simulink subsystem "WindGFLMpp"  (R2025b)
settings: Solver=VariableStepAuto  StartTime=0.0  StopTime=10.0  RelTol=1e-3
model mask{p=0, psim=0, Rs=0, Ld=0, Lq=0, Kdip_sm=0, Kdii_sm=0, Kqip_sm=0, Kqii_sm=0, airDensity=0, turbineRadius=0, pitch=0, TSR=0, cp=0, wt=0, rt=0, Inertia=0, Kp_dc=0, Ki_dc=0, Kdpi_g=0, Kdii_g=0, Kqpi_g=0, Kqii_g=0, blk=Enabled, slop=0, tst=0}
  mask prompts: p "Number of pole pairs"; psim "PMSM flux linkage"; Rs "Stator resistance (Ohms)"; Ld "Stator d-axis inductance (H)"; Lq "Stator q-axis inductance (H)"; Kdip_sm "d-axis proportional gain"; Kdii_sm "d-axis integral gain"; Kqip_sm "q-axis proportional gain"; Kqii_sm "q-axis integral gain"; airDensity "Air Density"; turbineRadius "Turbine radius"; pitch "Pitch angle vector"; cp "Power Coefficient (cp)"; wt "Wind velocity threshold"; rt "Rotational velocity threshold"; Inertia "Turbine Inertia (kgm^2)"; Kp_dc "Proportional gain"; Ki_dc "Integral gain"; Kdpi_g "d-axis proportional gain"; Kdii_g "d-axis integrall gain"; Kqpi_g "q-axis proportional gain"; Kqii_g "q-axis integral gain"; blk "Enable Black Start"; slop "Power Ramp Slope"; tst "Black Start time (sec)"
undefined symbols (not defined in the file): base, DiscIntNeverNeededParam, grid, mpptPower, mpptWindSpeed, Ts, windController, windInverter, windTurbine
libraries: nesl_utility x13, ee_lib x8, fl_lib x8, simulink x6, eeTransforms x4, eeGeneralControl x1, eePmsmCurrentController x1
settings Model: Creator=rajarshd  LastModifiedBy=rajarshd
settings OptimizationCC: ReuseModelBlockBuffer=off
settings RTWCC: GPUComputeCapability=3.5

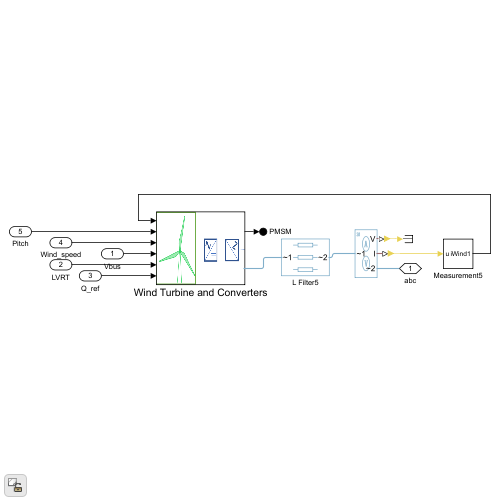
[thumbnail: Simulink's stored preview of the top-level diagram]
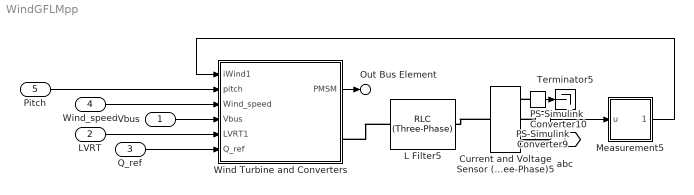
== system WindGFLMpp ==
  Vbus : Inport
  LVRT : Inport  Port=2
  Q_ref : Inport  Port=3
  Wind_speed : Inport  Port=4
  Pitch : Inport  Port=5
  Current and Voltage Sensor (Three-Phase)5 : ee_lib/Sensors & Transducers/Current and Voltage Sensor (Three-Phase)  vMeasurementType=ee.enum.vmeasurement.lg  outputUnit=ee.enum.unit.pu  SRated=base.mVA A*V  VRated=base.kV V  I_specify=off  I_priority=None  I=[0, 0, 0] A  I_nominal_specify=off  I_nominal_value=1  I_nominal_unit=A  V_specify=off  V_priority=None  V=[0, 0, 0] V  V_nominal_specify=off  V_nominal_value=1  V_nominal_unit=V
      settings: InternalSimscapePortConfiguration="{\"Bottom\":[],\"Left\":[{\"id\":\"N1\",\"label\":\"~1\",\"type\":\"foundation.electrical.three_phase\"}],\"Right\":[{\"id\":\"V_output\",\"label\":\"V\",\"type\":\"output\"},{\"id\":\"I_output\",\"label\":\"I\",\"type\":\"output\"},{\"id\":\"N2\",\"label\":\"~2\",\"type\":\"foundation.electrical.three_phase\"}],\"Top\":[]}"
  L Filter5 : ee_lib/Passive/RLC Assemblies/RLC (Three-Phase)  port_option=ee.enum.threePhasePort.composite  component_structure=ee.enum.rlc.structure.L  R=1e-3 Ohm  L=windInverter.l H  C=1e-6 F  R_parasitic=0 Ohm  G_parasitic=0 1/Ohm  IL_specify=off  IL_priority=High  IL=[0, 0, 0] A  IL_nominal_specify=off  IL_nominal_value=1  IL_nominal_unit=A  VC_specify=off  VC_priority=High  VC=[0, 0, 0] V  VC_nominal_specify=off  VC_nominal_value=1  VC_nominal_unit=V
      settings: InternalSimscapePortConfiguration="{\"Bottom\":[],\"Left\":[{\"id\":\"N1\",\"label\":\"~1\",\"type\":\"foundation.electrical.three_phase\"}],\"Right\":[{\"id\":\"N2\",\"label\":\"~2\",\"type\":\"foundation.electrical.three_phase\"}],\"Top\":[]}"
  Measurement5 : Subsystem
  PS-Simulink Converter10 : nesl_utility/PS-Simulink Converter  PhysicalDomain=network_engine_domain  SubClassName=ps_output  LeftPortType=input  RightPortType=output  PseudoPeriodic=off  Frequencies=[]  VectorFormat=inherit  Unit=inherit  AffineConversion=off
  PS-Simulink Converter9 : nesl_utility/PS-Simulink Converter  PhysicalDomain=network_engine_domain  SubClassName=ps_output  LeftPortType=input  RightPortType=output  PseudoPeriodic=off  Frequencies=[]  VectorFormat=inherit  Unit=inherit  AffineConversion=off
  Terminator5 : Terminator
  Wind Turbine and Converters : Subsystem
      mask Display: image('T4wind.png'); % Use "Edit Image" on toolstrip to change.
  abc : PMIOPort  Side=Right
  Out Bus Element : Outport  PortName=PMSM
  wires:
  PS-Simulink Converter10/1 -> Terminator5/1
  PS-Simulink Converter9/1 -> Measurement5/1(u)
  Wind_speed/1 -> Wind Turbine and Converters/3(Wind_speed)
  Wind Turbine and Converters/1(PMSM) -> Out Bus Element/1
  Vbus/1 -> Wind Turbine and Converters/4(Vbus)
  LVRT/1 -> Wind Turbine and Converters/5(LVRT1)
  Q_ref/1 -> Wind Turbine and Converters/6(Q_ref)
  Measurement5/1(iWind1) -> Wind Turbine and Converters/1(iWind1)
  Pitch/1 -> Wind Turbine and Converters/2(pitch)
  connections:
  PS-Simulink Converter9/LConn1 -- Current and Voltage Sensor (Three-Phase)5/RConn2
  PS-Simulink Converter10/LConn1 -- Current and Voltage Sensor (Three-Phase)5/RConn1
  L Filter5/LConn1 -- Wind Turbine and Converters/RConn1
  Current and Voltage Sensor (Three-Phase)5/LConn1 -- L Filter5/RConn1
  Current and Voltage Sensor (Three-Phase)5/RConn3 -- abc/RConn1

== system WindGFLMpp/Measurement5 ==
  u : Inport
  Low-Pass Filter (Discrete or Continuous) : eeGeneralControl/Low-Pass Filter (Discrete or Continuous)  K=1  T=2e-4  B=inf  A=-inf  init_option=Inherited from block input  x0=0  Ts=-1
  Out Bus Element : Outport  PortName=iWind1  Element=1
  wires:
  Low-Pass Filter (Discrete or Continuous)/1 -> Out Bus Element/1
  u/1 -> Low-Pass Filter (Discrete or Continuous)/1

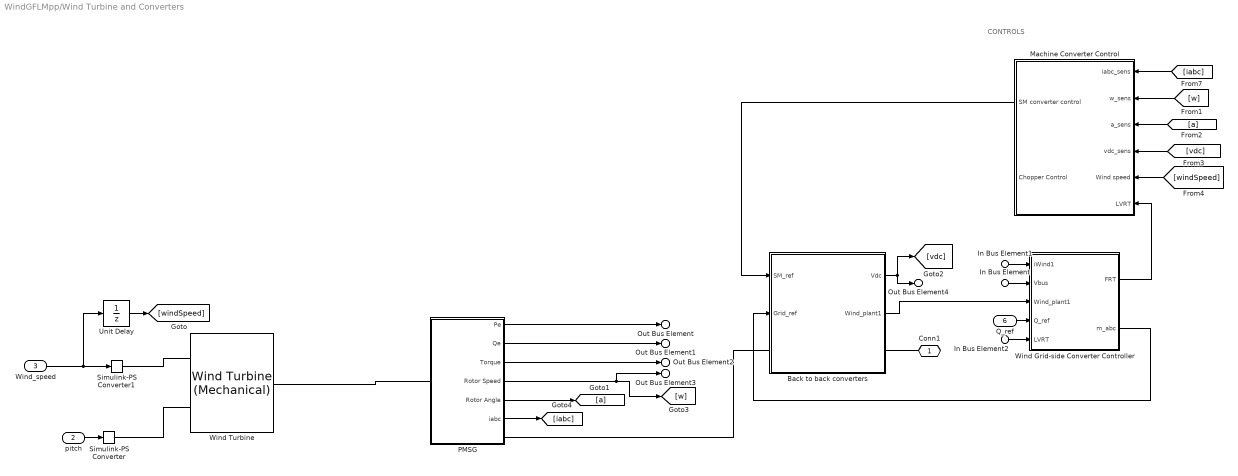
== system WindGFLMpp/Wind Turbine and Converters ==
  note: CONTROLS
  In Bus Element1 : Inport  PortName=iWind1
  pitch : Inport  Port=2
  Wind_speed : Inport  Port=3
  In Bus Element : Inport  Port=4  PortName=Vbus
  In Bus Element2 : Inport  Port=5  PortName=LVRT1
  Q_ref : Inport  Port=6
  Back to back converters : Subsystem
  Machine Converter Control : Subsystem
  PMSG : Subsystem
  Simulink-PS Converter : nesl_utility/Simulink-PS Converter  PhysicalDomain=network_engine_domain  SubClassName=ps_input  LeftPortType=input  RightPortType=output  PseudoPeriodic=off  Frequencies=[]  NoiseDistribution=none  NoiseParameters=[]  Unit=1  AffineConversion=off  FilteringAndDerivatives=provide  SimscapeFilterOrder=1  InputFilterTimeConstant=0.001  UdotUserProvided=0
  Simulink-PS Converter1 : nesl_utility/Simulink-PS Converter  PhysicalDomain=network_engine_domain  SubClassName=ps_input  LeftPortType=input  RightPortType=output  PseudoPeriodic=off  Frequencies=[]  NoiseDistribution=none  NoiseParameters=[]  Unit=1  AffineConversion=off  FilteringAndDerivatives=provide  SimscapeFilterOrder=1  InputFilterTimeConstant=0.001  UdotUserProvided=0
  Unit Delay : UnitDelay  SampleTime=-1  HasFrameUpgradeWarning=on
  Wind Grid-side Converter Controller : Subsystem
  "Wind Turbine " : ee_lib/Electromechanical/Wind Turbine (Mechanical)  R_rotor=turbineRadius m  pitch_TLU=pitch deg  lambda_TLU=TSR  Cp_TLU=cp  v_thr=wt m/s  w_thr=rt rad/s  rho_air=airDensity kg/m^3  includeInertia=true  J=Inertia kg*m^2  lam=0 N*m*s/rad  w_specify=off  w_priority=Low  w=2.262*2.5 rad/s  w_nominal_specify=off  w_nominal_value=1  w_nominal_unit=rad/s  t_specify=off  t_priority=None  t=0 N*m  t_nominal_specify=off  t_nominal_value=1  t_nominal_unit=N*m  Torque_specify=off  Torque_priority=None  Torque=0 N*m  Torque_nominal_specify=off  Torque_nominal_value=1  Torque_nominal_unit=N*m
      settings: InternalSimscapePortConfiguration="{\"Bottom\":[],\"Left\":[{\"id\":\"vWind\",\"label\":\"V\",\"type\":\"input\"},{\"id\":\"pitch\",\"label\":\"β\",\"type\":\"input\"}],\"Right\":[{\"id\":\"R\",\"label\":\"R\",\"type\":\"foundation.mechanical.rotational.rotational\"}],\"Top\":[]}"
  Conn1 : PMIOPort  Side=Right
  Out Bus Element : Outport  PortName=PMSM  Element=P
  Out Bus Element1 : Outport  PortName=PMSM  Element=Q
  Out Bus Element2 : Outport  PortName=PMSM  Element=Torque
  Out Bus Element3 : Outport  PortName=PMSM  Element=w_speed
  Out Bus Element4 : Outport  PortName=PMSM  Element=Vdc
  wires:
  Wind Grid-side Converter Controller/2(m_abc) -> Back to back converters/2(Grid_ref)
  Machine Converter Control/1(SM converter control) -> Back to back converters/1(SM_ref)
  In Bus Element2/1 -> Wind Grid-side Converter Controller/5(LVRT)
  Back to back converters/2(Wind_plant1) -> Wind Grid-side Converter Controller/3(Wind_plant1)
  Q_ref/1 -> Wind Grid-side Converter Controller/4(Q_ref)
  Wind Grid-side Converter Controller/1(FRT) -> Machine Converter Control/6(LVRT)
  In Bus Element/1 -> Wind Grid-side Converter Controller/2(Vbus)
  PMSG/1(Pe) -> Out Bus Element/1
  PMSG/5(Rotor Angle) -> [a]
  Back to back converters/1(Vdc) -> Out Bus Element4/1, [vdc]
  PMSG/6(iabc) -> [iabc]
  pitch/1 -> Simulink-PS Converter/1
  [windSpeed] -> Machine Converter Control/5(Wind speed)
  [w] -> Machine Converter Control/2(w_sens)
  [a] -> Machine Converter Control/3(a_sens)
  Wind_speed/1 -> Unit Delay/1, Simulink-PS Converter1/1
  [iabc] -> Machine Converter Control/1(iabc_sens)
  Unit Delay/1 -> [windSpeed]
  [vdc] -> Machine Converter Control/4(vdc_sens)
  In Bus Element1/1 -> Wind Grid-side Converter Controller/1(iWind1)
  PMSG/3(Torque) -> Out Bus Element2/1
  PMSG/2(Qe) -> Out Bus Element1/1
  PMSG/4(Rotor Speed) -> Out Bus Element3/1, [w]
  connections:
  PMSG/RConn1 -- Back to back converters/LConn1
  Conn1/RConn1 -- Back to back converters/RConn1
  "Wind Turbine "/LConn1 -- Simulink-PS Converter1/RConn1
  "Wind Turbine "/LConn2 -- Simulink-PS Converter/RConn1
  "Wind Turbine "/RConn1 -- PMSG/LConn1

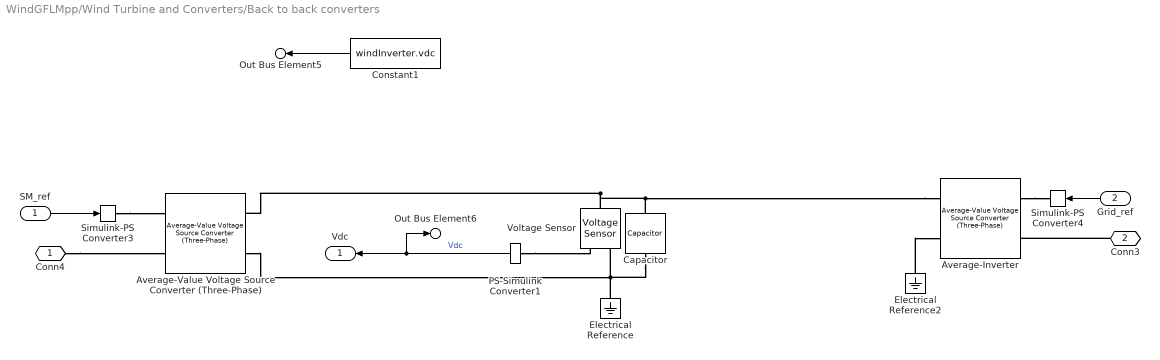
== system WindGFLMpp/Wind Turbine and Converters/Back to back converters ==
  SM_ref : Inport
  Grid_ref : Inport  Port=2
  Average-Inverter : ee_lib/Semiconductors & Converters/Converters/Average-Value Voltage Source Converter (Three-Phase)  port_option=ee.enum.threePhasePort.composite  frequency_option=ee.enum.converters.frequency.variable  input_option=ee.enum.converters.inputOption.ModWave  FRated=60 Hz  losses_parameterization=ee.enum.converters.losses.fixed  Pfixed=1 W  ks=0.01  kc1=1.7 V  kc2=0.01 Ohm  Ploss_vect=[100, 800, 1870, 3250, 4900] W  Irms_vect=[10, 100, 200, 300, 400] A  Vdc_nom=300 V  thermal_mass=30000 J/K  temperature_specify=off  temperature_priority=High  temperature=298.15 K  temperature_nominal_specify=off  temperature_nominal_value=1  temperature_nominal_unit=K
      settings: InternalSimscapePortConfiguration="{\"Bottom\":[],\"Left\":[{\"id\":\"ModWave\",\"label\":\"ModWave\",\"type\":\"input\"},{\"id\":\"N\",\"label\":\"~\",\"type\":\"foundation.electrical.three_phase\"}],\"Right\":[{\"id\":\"p\",\"label\":\"+\",\"type\":\"foundation.electrical.electrical\"},{\"id\":\"n\",\"label\":\"-\",\"type\":\"foundation.electrical.electrical\"}],\"Top\":[]}"
  Average-Value Voltage Source Converter (Three-Phase) : ee_lib/Semiconductors & Converters/Converters/Average-Value Voltage Source Converter (Three-Phase)  port_option=ee.enum.threePhasePort.composite  frequency_option=ee.enum.converters.frequency.variable  input_option=ee.enum.converters.inputOption.ModWave  FRated=60 Hz  losses_parameterization=ee.enum.converters.losses.fixed  Pfixed=1 W  ks=0.01  kc1=1.7 V  kc2=0.01 Ohm  Ploss_vect=[100, 800, 1870, 3250, 4900] W  Irms_vect=[10, 100, 200, 300, 400] A  Vdc_nom=300 V  thermal_mass=30000 J/K  temperature_specify=off  temperature_priority=High  temperature=298.15 K  temperature_nominal_specify=off  temperature_nominal_value=1  temperature_nominal_unit=K
      settings: InternalSimscapePortConfiguration="{\"Bottom\":[],\"Left\":[{\"id\":\"ModWave\",\"label\":\"ModWave\",\"type\":\"input\"},{\"id\":\"N\",\"label\":\"~\",\"type\":\"foundation.electrical.three_phase\"}],\"Right\":[{\"id\":\"p\",\"label\":\"+\",\"type\":\"foundation.electrical.electrical\"},{\"id\":\"n\",\"label\":\"-\",\"type\":\"foundation.electrical.electrical\"}],\"Top\":[]}"
  Capacitor : fl_lib/Electrical/Electrical Elements/Capacitor  c=windInverter.c F  r=0 Ohm  g=0 1/Ohm  i_specify=off  i_priority=None  i=0 A  i_nominal_specify=off  i_nominal_value=1  i_nominal_unit=A  v_specify=off  v_priority=None  v=0 V  v_nominal_specify=off  v_nominal_value=1  v_nominal_unit=V  vc_specify=on  vc_priority=Low  vc=windInverter.vdc V  vc_nominal_specify=off  vc_nominal_value=1  vc_nominal_unit=V
  Constant1 : Constant  Value=windInverter.vdc  SampleTime=Ts
  Electrical Reference : fl_lib/Electrical/Electrical Elements/Electrical Reference
  Electrical Reference2 : fl_lib/Electrical/Electrical Elements/Electrical Reference
  PS-Simulink Converter1 : nesl_utility/PS-Simulink Converter  PhysicalDomain=network_engine_domain  SubClassName=ps_output  LeftPortType=input  RightPortType=output  PseudoPeriodic=off  Frequencies=[]  VectorFormat=1-D array  Unit=V  AffineConversion=off
  Simulink-PS Converter3 : nesl_utility/Simulink-PS Converter  PhysicalDomain=network_engine_domain  SubClassName=ps_input  LeftPortType=input  RightPortType=output  PseudoPeriodic=off  Frequencies=[]  NoiseDistribution=none  NoiseParameters=[]  Unit=1  AffineConversion=off  FilteringAndDerivatives=provide  SimscapeFilterOrder=1  InputFilterTimeConstant=0.001  UdotUserProvided=0
  Simulink-PS Converter4 : nesl_utility/Simulink-PS Converter  PhysicalDomain=network_engine_domain  SubClassName=ps_input  LeftPortType=input  RightPortType=output  PseudoPeriodic=off  Frequencies=[]  NoiseDistribution=none  NoiseParameters=[]  Unit=1  AffineConversion=off  FilteringAndDerivatives=provide  SimscapeFilterOrder=1  InputFilterTimeConstant=0.001  UdotUserProvided=0
  Voltage Sensor : fl_lib/Electrical/Electrical Sensors/Voltage Sensor
  Conn4 : PMIOPort  Side=Left
  Conn3 : PMIOPort  Port=2  Side=Right
  Vdc : Outport
  Out Bus Element6 : Outport  Port=2  PortName=Wind_plant1  Element=Vdc_measured
  Out Bus Element5 : Outport  Port=2  PortName=Wind_plant1  Element=windInverter.vdc
  wires:
  Constant1/1 -> Out Bus Element5/1
  SM_ref/1 -> Simulink-PS Converter3/1
  Grid_ref/1 -> Simulink-PS Converter4/1
  PS-Simulink Converter1/1 -> Vdc/1, Out Bus Element6/1  "Vdc"
  connections:
  Conn3/RConn1 -- Average-Inverter/LConn2
  Simulink-PS Converter3/RConn1 -- Average-Value Voltage Source Converter (Three-Phase)/LConn1
  Average-Inverter/LConn1 -- Simulink-PS Converter4/RConn1
  Conn4/RConn1 -- Average-Value Voltage Source Converter (Three-Phase)/LConn2
  Average-Value Voltage Source Converter (Three-Phase)/RConn2 -- Electrical Reference/LConn1 -- Capacitor/RConn1 -- Voltage Sensor/RConn2
  Electrical Reference2/LConn1 -- Average-Inverter/RConn2
  Average-Inverter/RConn1 -- Capacitor/LConn1 -- Average-Value Voltage Source Converter (Three-Phase)/RConn1 -- Voltage Sensor/LConn1
  PS-Simulink Converter1/LConn1 -- Voltage Sensor/RConn1

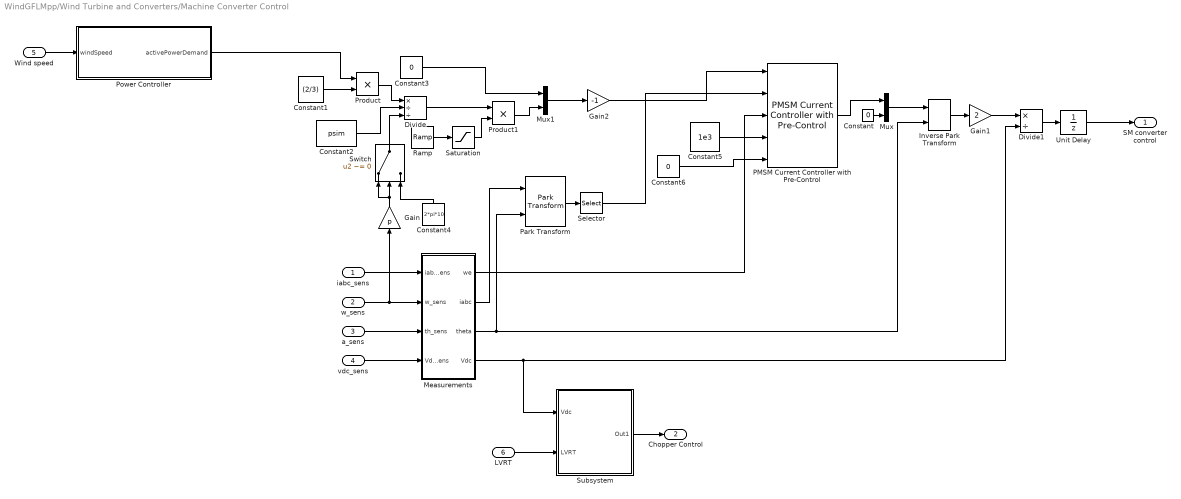
== system WindGFLMpp/Wind Turbine and Converters/Machine Converter Control ==
  iabc_sens : Inport
  w_sens : Inport  Port=2
  a_sens : Inport  Port=3
  vdc_sens : Inport  Port=4
  Wind speed : Inport  Port=5
  LVRT : Inport  Port=6
  Constant : Constant  Value=0  SampleTime=-1
  Constant1 : Constant  Value=(2/3)
  Constant2 : Constant  Value=psim
  Constant3 : Constant  Value=0
  Constant4 : Constant  Value=2*pi*10
  Constant5 : Constant  Value=1e3  VectorParams1D=off  SampleTime=-1
  Constant6 : Constant  Value=0
  Divide : Product  Inputs=*//
  Divide1 : Product  Inputs=*/
  Gain : Gain  Gain=p
  Gain1 : Gain  Gain=2
  Gain2 : Gain  Gain=-1
  Inverse Park Transform : eeTransforms/Inverse Park Transform  AxisAlignment=Q-axis  PowerInvariant=off
  Measurements : Subsystem
  Mux : Mux  Inputs=2
  Mux1 : Mux  Inputs=2
  PMSM Current Controller with Pre-Control : eePmsmCurrentController/PMSM Current Controller with Pre-Control  Kp_id=Kdip_sm  Ki_id=Kdii_sm  Kaw_id=0  Kp_iq=Kqip_sm  Ki_iq=Kqii_sm  Kaw_iq=0  Ts=-1  Tsd=0.001  AxisPrio=Q-axis  ActZC=off  ActFF=on  idVect=[-1, 0, 1]  iqVect=[-2000, 0, 2000]  LdMatrix=Ld* ones(3, 3)  LqMatrix=Lq* ones(3, 3)  psimMatrix=psim * ones(3, 3)
  Park Transform : eeTransforms/Park Transform  AxisAlignment=Q-axis  PowerInvariant=off
  Power Controller : Subsystem
  Product : Product
  Product1 : Product
  Ramp : simulink/Sources/Ramp  slope=slop  start=tst  InitialOutput=blk
  Saturation : Saturate  UpperLimit=1  LowerLimit=0
  Selector : Selector  InputPortWidth=3  IndexOptions=Index vector (dialog)  Indices=[1 2]  OutputSizes=1
  Subsystem : Subsystem
  Switch : Switch  Criteria=u2 ~= 0  SaturateOnIntegerOverflow=off  InputSameDT=off
  Unit Delay : UnitDelay  SampleTime=-1  HasFrameUpgradeWarning=on
  SM converter control : Outport  VectorParamsAs1DForOutWhenUnconnected=off
  Chopper Control : Outport  Port=2
  wires:
  Saturation/1 -> Product1/2
  Product1/1 -> Mux1/2
  Divide/1 -> Product1/1
  Power Controller/1(activePowerDemand) -> Product/1
  Ramp/1 -> Saturation/1
  Wind speed/1 -> Power Controller/1(windSpeed)
  Subsystem/1(Out1) -> Chopper Control/1
  LVRT/1 -> Subsystem/2(LVRT)
  PMSM Current Controller with Pre-Control/1 -> Mux/1
  Gain2/1 -> PMSM Current Controller with Pre-Control/1
  Constant4/1 -> Switch/3
  Switch/1 -> Divide/3
  Gain/1 -> Switch/2, Switch/1
  Constant1/1 -> Product/2
  Product/1 -> Divide/1
  Mux1/1 -> Gain2/1
  Constant3/1 -> Mux1/1
  Constant2/1 -> Divide/2
  Constant6/1 -> PMSM Current Controller with Pre-Control/5
  Constant5/1 -> PMSM Current Controller with Pre-Control/4
  Gain1/1 -> Divide1/1
  Selector/1 -> PMSM Current Controller with Pre-Control/2
  Park Transform/1 -> Selector/1
  Measurements/3(theta) -> Inverse Park Transform/2, Park Transform/2
  Measurements/2(iabc) -> Park Transform/1
  Unit Delay/1 -> SM converter control/1
  Constant/1 -> Mux/2
  Mux/1 -> Inverse Park Transform/1
  Inverse Park Transform/1 -> Gain1/1
  a_sens/1 -> Measurements/3(th_sens)
  iabc_sens/1 -> Measurements/1(iabc_sens)
  Measurements/1(we) -> PMSM Current Controller with Pre-Control/3
  w_sens/1 -> Measurements/2(w_sens), Gain/1
  vdc_sens/1 -> Measurements/4(Vdc_sens)
  Divide1/1 -> Unit Delay/1
  Measurements/4(Vdc) -> Divide1/2, Subsystem/1(Vdc)

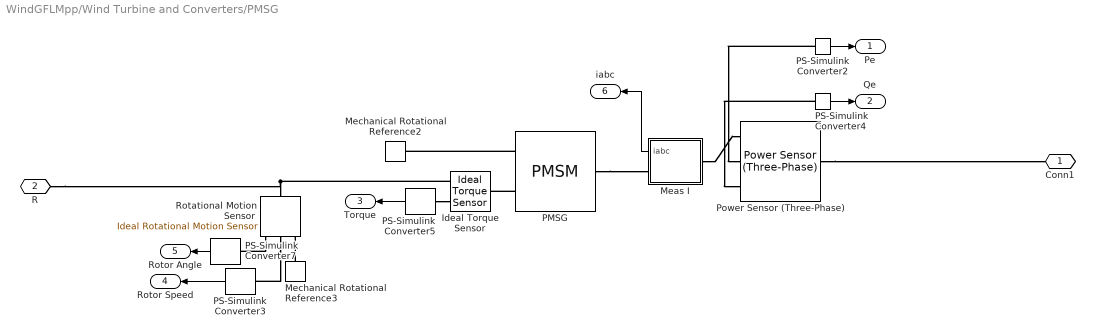
== system WindGFLMpp/Wind Turbine and Converters/PMSG ==
  Ideal Torque Sensor : fl_lib/Mechanical/Mechanical Sensors/Ideal Torque Sensor
  Meas I : Subsystem
  Mechanical Rotational Reference2 : fl_lib/Mechanical/Rotational Elements/Mechanical Rotational Reference
  Mechanical Rotational Reference3 : fl_lib/Mechanical/Rotational Elements/Mechanical Rotational Reference
  PMSG : ee_lib/Electromechanical/Permanent Magnet/PMSM  port_option=ee.enum.threePhasePort.composite  winding_type=ee.enum.statorconnection.wye  machine_param=ee.enum.pmsm.parameterization.constant  nPolePairs=p  pmflux_param=ee.enum.pmflux.fluxlinkage  pm_flux_linkage=psim Wb  torque_constant=0.18 N*m/A  back_emf_constant=0.18 V*s/rad  stator_param=ee.enum.statorparam.LdLqL0  Ld=Ld H  Lq=Lq H  idVec=[-200, 0, 200] A  iqVec=[-200, 0, 200] A  LdMatrix=0.0002 * ones(3, 3) H  LqMatrix=0.0002 * ones(3, 3) H  PmMatrix=0.1 * ones(3, 3) Wb  ktMatrix=0.18 * ones(3, 3) N*m/A  keMatrix=0.18 * ones(3, 3) V*s/rad  L0=0.00016 H  Ls=0.0002 H  Lm=-0.00002 H  Ms=0.00002 H  Rs=Rs Ohm  zero_sequence=ee.enum.park.zerosequence.exclude  axes_param=ee.enum.rotorangle.qaxis  loss_param=ee.enum.ironloss.none  losses_oc=[0, 0, 0] W  losses_sc=[0, 0, 0] W  f_losses=60 Hz  Isc_losses=95 A  J=200 kg*m^2  lam=1e-4 N*m*s/rad  i_d_specify=off  i_d_priority=None  i_d=0 A  i_d_nominal_specify=off  i_d_nominal_value=1  i_d_nominal_unit=A  i_q_specify=off  i_q_priority=None  i_q=0 A  i_q_nominal_specify=off  i_q_nominal_value=1  i_q_nominal_unit=A  torque_specify=off  torque_priority=None  torque=0 N*m  torque_nominal_specify=off  torque_nominal_value=1  torque_nominal_unit=N*m  angular_velocity_specify=on  angular_velocity_priority=High  angular_velocity=2.26 rad/s  angular_velocity_nominal_specify=off  angular_velocity_nominal_value=1  angular_velocity_nominal_unit=rpm  angular_position_specify=off  angular_position_priority=High  angular_position=0 deg  angular_position_nominal_specify=off  angular_position_nominal_value=1  angular_position_nominal_unit=deg  alpha=3.93e-3 1/K  alpha_flux=-0.001 1/K  Tmeas=298.15 K  stator_thermal_mass=100 J/K  rotor_thermal_mass=200 J/K  Rm_percent_rotor=90  Rd_percent_rotor=30  temperatureA_specify=off  temperatureA_priority=High  temperatureA=25 degC  temperatureA_nominal_specify=off  temperatureA_nominal_value=1  temperatureA_nominal_unit=degC  temperatureB_specify=off  temperatureB_priority=High  temperatureB=25 degC  temperatureB_nominal_specify=off  temperatureB_nominal_value=1  temperatureB_nominal_unit=degC  temperatureC_specify=off  temperatureC_priority=High  temperatureC=25 degC  temperatureC_nominal_specify=off  temperatureC_nominal_value=1  temperatureC_nominal_unit=degC  temperatureR_specify=off  temperatureR_priority=High  temperatureR=25 degC  temperatureR_nominal_specify=off  temperatureR_nominal_value=1  temperatureR_nominal_unit=degC
      settings: InternalSimscapePortConfiguration="{\"Bottom\":[],\"Left\":[{\"id\":\"N\",\"label\":\"~\",\"type\":\"foundation.electrical.three_phase\"}],\"Right\":[{\"id\":\"R\",\"label\":\"R\",\"type\":\"foundation.mechanical.rotational.rotational\"},{\"id\":\"C\",\"label\":\"C\",\"type\":\"foundation.mechanical.rotational.rotational\"}],\"Top\":[]}"
  PS-Simulink Converter2 : nesl_utility/PS-Simulink Converter  PhysicalDomain=network_engine_domain  SubClassName=ps_output  LeftPortType=input  RightPortType=output  PseudoPeriodic=off  Frequencies=[]  VectorFormat=inherit  Unit=inherit  AffineConversion=off
  PS-Simulink Converter3 : nesl_utility/PS-Simulink Converter  PhysicalDomain=network_engine_domain  SubClassName=ps_output  LeftPortType=input  RightPortType=output  PseudoPeriodic=off  Frequencies=[]  VectorFormat=1-D array  Unit=rad/s  AffineConversion=off
  PS-Simulink Converter4 : nesl_utility/PS-Simulink Converter  PhysicalDomain=network_engine_domain  SubClassName=ps_output  LeftPortType=input  RightPortType=output  PseudoPeriodic=off  Frequencies=[]  VectorFormat=inherit  Unit=inherit  AffineConversion=off
  PS-Simulink Converter5 : nesl_utility/PS-Simulink Converter  PhysicalDomain=network_engine_domain  SubClassName=ps_output  LeftPortType=input  RightPortType=output  PseudoPeriodic=off  Frequencies=[]  VectorFormat=1-D array  Unit=N*m  AffineConversion=off
  PS-Simulink Converter7 : nesl_utility/PS-Simulink Converter  PhysicalDomain=network_engine_domain  SubClassName=ps_output  LeftPortType=input  RightPortType=output  PseudoPeriodic=off  Frequencies=[]  VectorFormat=1-D array  Unit=rad  AffineConversion=off
  Power Sensor (Three-Phase) : ee_lib/Sensors & Transducers/Power Sensor (Three-Phase)  load_type=ee.enum.passive.type_balanced.balanced  f0=60 Hz
      settings: InternalSimscapePortConfiguration="{\"Bottom\":[],\"Left\":[{\"id\":\"N1\",\"label\":\"~1\",\"type\":\"foundation.electrical.three_phase\"}],\"Right\":[{\"id\":\"N2\",\"label\":\"~2\",\"type\":\"foundation.electrical.three_phase\"}],\"Top\":[{\"id\":\"Pm\",\"label\":\"P\",\"type\":\"output\"},{\"id\":\"Qm\",\"label\":\"Q\",\"type\":\"output\"}]}"
  Rotational Motion Sensor : fl_lib/Mechanical/Mechanical Sensors/Ideal Rotational Motion Sensor  reference=foundation.enum.MeasurementReference.difference  acceleration_port=false  velocity_port=true  position_port=true  wrap_angle=simscape.enum.onoff.off  offset=0 deg
  Conn1 : PMIOPort  Side=Right
  R : PMIOPort  Port=2  Side=Left
  Pe : Outport
  Qe : Outport  Port=2
  Torque : Outport  Port=3
  Rotor Speed : Outport  Port=4
  Rotor Angle : Outport  Port=5
  iabc : Outport  Port=6
  wires:
  PS-Simulink Converter5/1 -> Torque/1
  PS-Simulink Converter4/1 -> Qe/1
  PS-Simulink Converter2/1 -> Pe/1
  PS-Simulink Converter7/1 -> Rotor Angle/1
  PS-Simulink Converter3/1 -> Rotor Speed/1
  Meas I/1(iabc) -> iabc/1
  connections:
  PMSG/LConn1 -- Meas I/RConn1
  Meas I/LConn1 -- Power Sensor (Three-Phase)/LConn1
  Power Sensor (Three-Phase)/RConn1 -- Conn1/RConn1
  PS-Simulink Converter5/LConn1 -- Ideal Torque Sensor/RConn2
  PS-Simulink Converter2/LConn1 -- Power Sensor (Three-Phase)/LConn2
  PS-Simulink Converter4/LConn1 -- Power Sensor (Three-Phase)/LConn3
  Mechanical Rotational Reference3/LConn1 -- Rotational Motion Sensor/RConn1
  PMSG/RConn1 -- Ideal Torque Sensor/LConn1
  Rotational Motion Sensor/RConn3 -- PS-Simulink Converter7/LConn1
  Rotational Motion Sensor/RConn2 -- PS-Simulink Converter3/LConn1
  R/RConn1 -- Ideal Torque Sensor/RConn1 -- Rotational Motion Sensor/LConn1
  PMSG/RConn2 -- Mechanical Rotational Reference2/LConn1

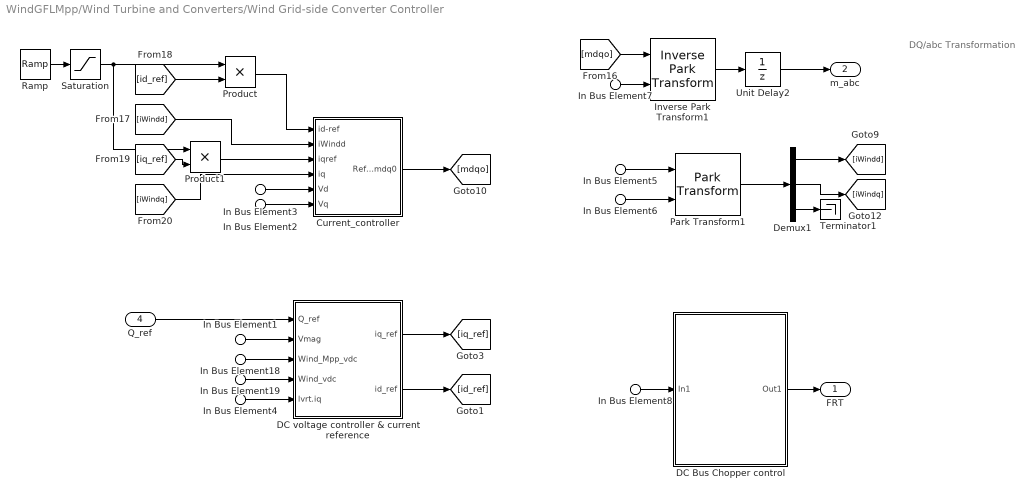
== system WindGFLMpp/Wind Turbine and Converters/Wind Grid-side Converter Controller ==
  note: DQ/abc Transformation
  In Bus Element5 : Inport  PortName=iWind1  Element=1
  In Bus Element3 : Inport  Port=2  PortName=Vbus  Element=Vd
  In Bus Element2 : Inport  Port=2  PortName=Vbus  Element=Vq
  In Bus Element6 : Inport  Port=2  PortName=Vbus  Element=Theta
  In Bus Element7 : Inport  Port=2  PortName=Vbus  Element=Theta
  In Bus Element1 : Inport  Port=2  PortName=Vbus  Element=Vmag
  In Bus Element8 : Inport  Port=2  PortName=Vbus  Element=Vmag
  In Bus Element18 : Inport  Port=3  PortName=Wind_plant1  Element=Vdc_measured
  In Bus Element19 : Inport  Port=3  PortName=Wind_plant1  Element=windInverter.vdc
  Q_ref : Inport  Port=4
  In Bus Element4 : Inport  Port=5  PortName=LVRT
  Current_controller : Subsystem
  "DC Bus Chopper control " : Subsystem
  DC voltage controller & current reference : Subsystem
  Demux1 : Demux  Outputs=3
  Inverse Park Transform1 : eeTransforms/Inverse Park Transform  AxisAlignment=Q-axis  PowerInvariant=off
  Park Transform1 : eeTransforms/Park Transform  AxisAlignment=Q-axis  PowerInvariant=off
  Product : Product
  Product1 : Product
  Ramp : simulink/Sources/Ramp  slope=slop  start=tst  InitialOutput=blk
  Saturation : Saturate  UpperLimit=1
  Terminator1 : Terminator
  Unit Delay2 : UnitDelay  SampleTime=Ts  HasFrameUpgradeWarning=on
  FRT : Outport
  m_abc : Outport  Port=2
  wires:
  Product1/1 -> Current_controller/3(iqref)
  [iq_ref] -> Product1/2
  [iWindd] -> Current_controller/2(iWindd)
  Product/1 -> Current_controller/1(id-ref)
  [id_ref] -> Product/2
  Saturation/1 -> Product/1, Product1/1
  Ramp/1 -> Saturation/1
  "DC Bus Chopper control "/1(Out1) -> FRT/1
  In Bus Element8/1 -> "DC Bus Chopper control "/1(In1)
  Q_ref/1 -> DC voltage controller & current reference/1(Q_ref)
  DC voltage controller & current reference/2(id_ref) -> [id_ref]
  DC voltage controller & current reference/1(iq_ref) -> [iq_ref]
  In Bus Element19/1 -> DC voltage controller & current reference/4(Wind_vdc)
  In Bus Element18/1 -> DC voltage controller & current reference/3(Wind_Mpp_vdc)
  In Bus Element4/1 -> DC voltage controller & current reference/5(lvrt.iq)
  In Bus Element1/1 -> DC voltage controller & current reference/2(Vmag)
  In Bus Element5/1 -> Park Transform1/1
  In Bus Element7/1 -> Inverse Park Transform1/2
  In Bus Element6/1 -> Park Transform1/2
  [iWindq] -> Current_controller/4(iq)
  In Bus Element3/1 -> Current_controller/5(Vd)
  Park Transform1/1 -> Demux1/1
  [mdqo] -> Inverse Park Transform1/1
  Demux1/3 -> Terminator1/1
  Demux1/1 -> [iWindd]
  Unit Delay2/1 -> m_abc/1
  Demux1/2 -> [iWindq]
  Inverse Park Transform1/1 -> Unit Delay2/1
  Current_controller/1(Refrence_mdq0) -> [mdqo]
  In Bus Element2/1 -> Current_controller/6(Vq)

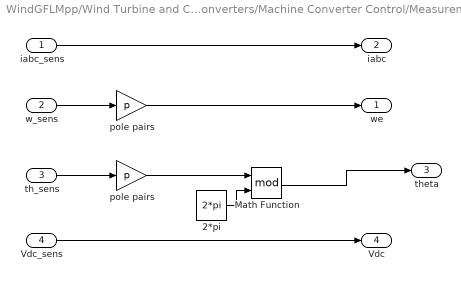
== system WindGFLMpp/Wind Turbine and Converters/Machine Converter Control/Measurements ==
  iabc_sens : Inport
  w_sens : Inport  Port=2
  th_sens : Inport  Port=3
  Vdc_sens : Inport  Port=4
  2*pi : Constant  Value=2*pi  SampleTime=-1
  Math Function : Math  Operator=mod  SignedPower=on
  pole pairs : Gain  Gain=p
  "pole pairs " : Gain  Gain=p
  we : Outport  VectorParamsAs1DForOutWhenUnconnected=off
  iabc : Outport  Port=2  VectorParamsAs1DForOutWhenUnconnected=off
  theta : Outport  Port=3  VectorParamsAs1DForOutWhenUnconnected=off
  Vdc : Outport  Port=4  VectorParamsAs1DForOutWhenUnconnected=off
  wires:
  Math Function/1 -> theta/1
  Vdc_sens/1 -> Vdc/1
  "pole pairs "/1 -> Math Function/1
  th_sens/1 -> "pole pairs "/1
  2*pi/1 -> Math Function/2
  pole pairs/1 -> we/1
  iabc_sens/1 -> iabc/1
  w_sens/1 -> pole pairs/1

== system WindGFLMpp/Wind Turbine and Converters/Machine Converter Control/Power Controller ==
  windSpeed : Inport
  Derating Control : Subsystem
  Greater than : simulink/Logic and Bit Operations/Compare To Constant  relop=>  const=windTurbine.vWindRated  OutDataTypeStr=boolean
  Less than or equal to : simulink/Logic and Bit Operations/Compare To Constant  relop=<=  const=windTurbine.vWindRated  OutDataTypeStr=boolean
  Limiter Function Power Demand : Subsystem
  MPPT Control : Subsystem
  activePowerDemand : Outport
  wires:
  Limiter Function Power Demand/1(activePowerDemand) -> activePowerDemand/1
  Derating Control/1(activePowerDemand) -> Limiter Function Power Demand/2(activePowerDemandDerating)
  MPPT Control/1(activePowerDemand) -> Limiter Function Power Demand/1(activePowerDemandMPPT)
  Greater than/1 -> Derating Control/Enable
  Less than or equal to/1 -> MPPT Control/Enable
  windSpeed/1 -> MPPT Control/1(windSpeed), Less than or equal to/1, Greater than/1

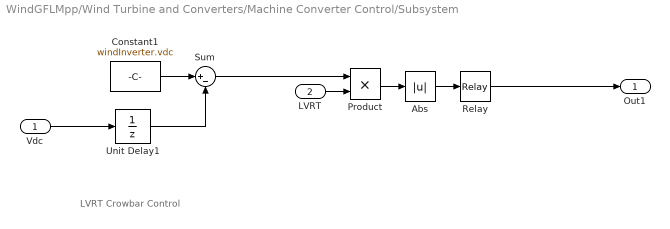
== system WindGFLMpp/Wind Turbine and Converters/Machine Converter Control/Subsystem ==
  note: LVRT Crowbar Control
  Vdc : Inport
  LVRT : Inport  Port=2
  Abs : Abs  SaturateOnIntegerOverflow=off
  Constant1 : Constant  Value=windInverter.vdc
  Product : Product
  Relay : Relay  OnSwitchValue=0.01001*windInverter.vdc  OffSwitchValue=0.01*windInverter.vdc
  Sum : Sum  Inputs=|+-
  Unit Delay1 : UnitDelay  SampleTime=-1  HasFrameUpgradeWarning=on
  Out1 : Outport
  wires:
  Relay/1 -> Out1/1
  Product/1 -> Abs/1
  LVRT/1 -> Product/2
  Unit Delay1/1 -> Sum/2
  Abs/1 -> Relay/1
  Sum/1 -> Product/1
  Vdc/1 -> Unit Delay1/1
  Constant1/1 -> Sum/1

== system WindGFLMpp/Wind Turbine and Converters/PMSG/Meas I ==
  Current Sensor : ee_lib/Sensors & Transducers/Current Sensor (Three-Phase)
  PS-Simulink Converter : nesl_utility/PS-Simulink Converter  PhysicalDomain=network_engine_domain  SubClassName=ps_output  LeftPortType=input  RightPortType=output  PseudoPeriodic=off  Frequencies=[]  VectorFormat=1-D array  Unit=A  AffineConversion=off
  1 : PMIOPort  Side=Left
  2 : PMIOPort  Port=2  Side=Right
  iabc : Outport
  wires:
  PS-Simulink Converter/1 -> iabc/1
  connections:
  Current Sensor/RConn2 -- 2/RConn1
  Current Sensor/LConn1 -- 1/RConn1
  Current Sensor/RConn1 -- PS-Simulink Converter/LConn1

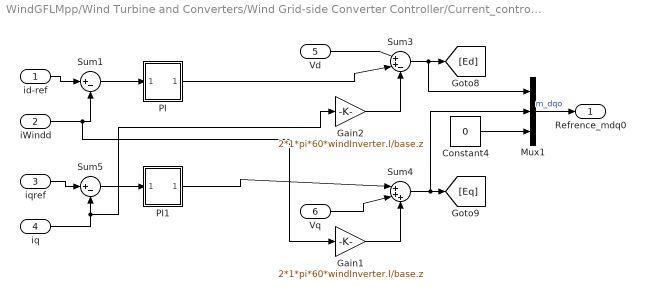
== system WindGFLMpp/Wind Turbine and Converters/Wind Grid-side Converter Controller/Current_controller ==
  id-ref : Inport
  iWindd : Inport  Port=2
  iqref : Inport  Port=3
  iq : Inport  Port=4
  Vd : Inport  Port=5
  Vq : Inport  Port=6
  Constant4 : Constant  Value=0
  Gain1 : Gain  Gain=2*1*pi*60*windInverter.l/base.z
  Gain2 : Gain  Gain=2*1*pi*60*windInverter.l/base.z
  Mux1 : Mux  Inputs=3
  PI : Subsystem
  PI1 : Subsystem
  Sum1 : Sum  Inputs=|+-
  Sum3 : Sum  Inputs=|++-
  Sum4 : Sum  Inputs=|+++
  Sum5 : Sum  Inputs=|+-
  Refrence_mdq0 : Outport
  wires:
  Mux1/1 -> Refrence_mdq0/1  "m_dqo"
  Sum4/1 -> [Eq], Mux1/2
  PI1/1(Out2) -> Sum4/1
  iqref/1 -> Sum5/1
  Sum5/1 -> PI1/1(Input)
  Constant4/1 -> Mux1/3
  Vd/1 -> Sum3/1
  Sum1/1 -> PI/1(Input)
  iq/1 -> Sum5/2, Gain2/1
  Vq/1 -> Sum4/2
  Gain1/1 -> Sum4/3
  id-ref/1 -> Sum1/1
  iWindd/1 -> Sum1/2, Gain1/1
  Gain2/1 -> Sum3/3
  Sum3/1 -> [Ed], Mux1/1
  PI/1(Out2) -> Sum3/2

== system WindGFLMpp/Wind Turbine and Converters/Wind Grid-side Converter Controller/DC Bus Chopper control  ==
  note: LVRT Detection
  In1 : Inport
  Constant1 : Constant
  Constant2 : Constant  Value=0
  Switch : Switch  Criteria=u2 > Threshold  Threshold=0.9  SaturateOnIntegerOverflow=off  InputSameDT=off
  Unit Delay : UnitDelay  SampleTime=-1  HasFrameUpgradeWarning=on
  Out1 : Outport
  wires:
  Unit Delay/1 -> Switch/2
  In1/1 -> Unit Delay/1
  Constant2/1 -> Switch/1
  Constant1/1 -> Switch/3
  Switch/1 -> Out1/1

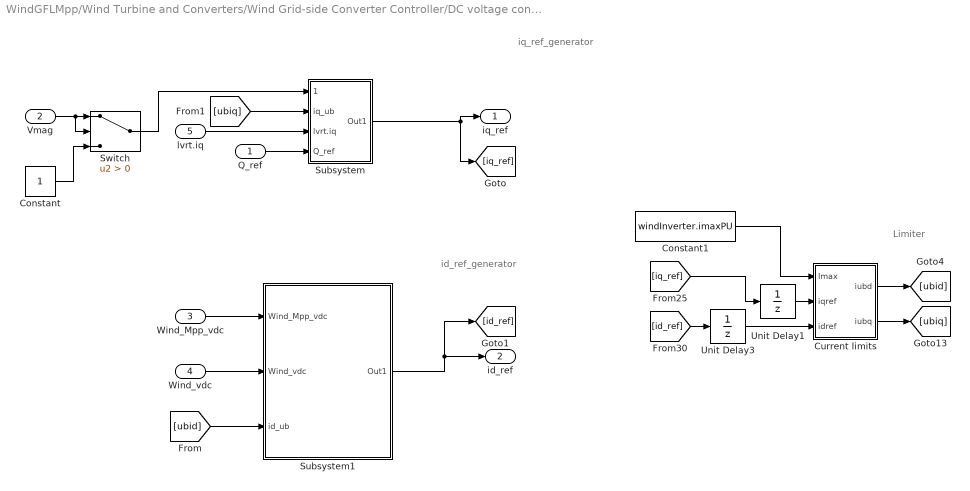
== system WindGFLMpp/Wind Turbine and Converters/Wind Grid-side Converter Controller/DC voltage controller & current reference ==
  note: id_ref_generator
  note: iq_ref_generator
  note: Limiter
  Q_ref : Inport
  Vmag : Inport  Port=2
  Wind_Mpp_vdc : Inport  Port=3
  Wind_vdc : Inport  Port=4
  lvrt.iq : Inport  Port=5
  Constant : Constant
  Constant1 : Constant  Value=windInverter.imaxPU
  Current limits : Subsystem
  Subsystem : Subsystem
  Subsystem1 : Subsystem
  Switch : Switch  Criteria=u2 > Threshold  SaturateOnIntegerOverflow=off  InputSameDT=off
  Unit Delay1 : UnitDelay  SampleTime=Ts  HasFrameUpgradeWarning=on
  Unit Delay3 : UnitDelay  SampleTime=Ts  HasFrameUpgradeWarning=on
  iq_ref : Outport
  id_ref : Outport  Port=2
  wires:
  Constant/1 -> Switch/3
  Switch/1 -> Subsystem/1(V_mag)
  Vmag/1 -> Switch/1, Switch/2
  lvrt.iq/1 -> Subsystem/3(lvrt.iq)
  [ubiq] -> Subsystem/2(iq_ub)
  [ubid] -> Subsystem1/3(id_ub)
  Subsystem/1(Out1) -> iq_ref/1, [iq_ref]
  Wind_vdc/1 -> Subsystem1/2(Wind_vdc)
  Wind_Mpp_vdc/1 -> Subsystem1/1(Wind_Mpp_vdc)
  Subsystem1/1(Out1) -> id_ref/1, [id_ref]
  Q_ref/1 -> Subsystem/4(Q_ref)
  Unit Delay3/1 -> Current limits/3(idref)
  [id_ref] -> Unit Delay3/1
  Unit Delay1/1 -> Current limits/2(iqref)
  Constant1/1 -> Current limits/1(Imax)
  Current limits/1(iubd) -> [ubid]
  Current limits/2(iubq) -> [ubiq]
  [iq_ref] -> Unit Delay1/1

== system WindGFLMpp/Wind Turbine and Converters/Machine Converter Control/Power Controller/Derating Control ==
  Enable : EnablePort  StatesWhenEnabling=reset
  Constant : Constant  Value=windTurbine.turbineRatedPower
  MW to W : Gain  Gain=1e6
  activePowerDemand : Outport
  wires:
  Constant/1 -> MW to W/1
  MW to W/1 -> activePowerDemand/1

== system WindGFLMpp/Wind Turbine and Converters/Machine Converter Control/Power Controller/Limiter Function Power Demand ==
  activePowerDemandMPPT : Inport
  activePowerDemandDerating : Inport  Port=2
  Merge : Merge
  activePowerDemand : Outport
  wires:
  Merge/1 -> activePowerDemand/1
  activePowerDemandDerating/1 -> Merge/2
  activePowerDemandMPPT/1 -> Merge/1

== system WindGFLMpp/Wind Turbine and Converters/Machine Converter Control/Power Controller/MPPT Control ==
  windSpeed : Inport
  Enable : EnablePort  StatesWhenEnabling=reset
  MW to W : Gain  Gain=1e6
  mpptActivePowerDemand : Lookup_n-D  NumberOfTableDimensions=1  BreakpointsForDimension1=mpptWindSpeed  Table=mpptPower  InternalRulePriority=Speed  RndMeth=Simplest
  activePowerDemand : Outport
  wires:
  MW to W/1 -> activePowerDemand/1
  windSpeed/1 -> mpptActivePowerDemand/1
  mpptActivePowerDemand/1 -> MW to W/1

== system WindGFLMpp/Wind Turbine and Converters/Wind Grid-side Converter Controller/Current_controller/PI ==
  Input : Inport
  Discrete-Time Integrator : DiscreteIntegrator  gainval=Kdii_g  SampleTime=grid.sensorTime  ICPrevOutput=DiscIntNeverNeededParam  ICPrevScaledInput=DiscIntNeverNeededParam
  Gain1 : Gain  Gain=Kdpi_g
  Sum1 : Sum  Inputs=|++
  Unit Delay : UnitDelay  SampleTime=grid.sensorTime  HasFrameUpgradeWarning=on
  Out2 : Outport
  wires:
  Input/1 -> Discrete-Time Integrator/1, Gain1/1
  Gain1/1 -> Unit Delay/1
  Unit Delay/1 -> Sum1/2
  Sum1/1 -> Out2/1
  Discrete-Time Integrator/1 -> Sum1/1

== system WindGFLMpp/Wind Turbine and Converters/Wind Grid-side Converter Controller/Current_controller/PI1 ==
  Input : Inport
  Discrete-Time Integrator : DiscreteIntegrator  gainval=Kqii_g  SampleTime=grid.sensorTime  ICPrevOutput=DiscIntNeverNeededParam  ICPrevScaledInput=DiscIntNeverNeededParam
  Gain1 : Gain  Gain=Kqpi_g
  Sum1 : Sum  Inputs=|++
  Unit Delay : UnitDelay  SampleTime=grid.sensorTime  HasFrameUpgradeWarning=on
  Out2 : Outport
  wires:
  Input/1 -> Discrete-Time Integrator/1, Gain1/1
  Gain1/1 -> Unit Delay/1
  Unit Delay/1 -> Sum1/2
  Sum1/1 -> Out2/1
  Discrete-Time Integrator/1 -> Sum1/1

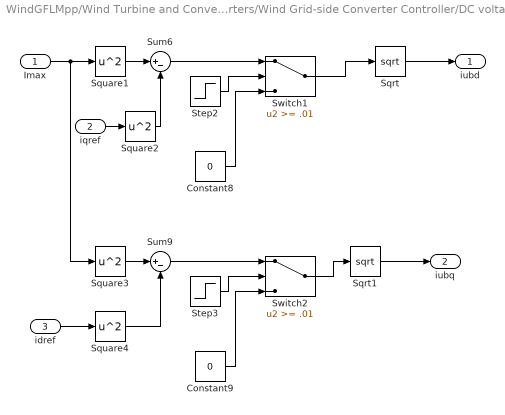
== system WindGFLMpp/Wind Turbine and Converters/Wind Grid-side Converter Controller/DC voltage controller & current reference/Current limits ==
  Imax : Inport
  iqref : Inport  Port=2
  idref : Inport  Port=3
  Constant8 : Constant  Value=0
  Constant9 : Constant  Value=0
  Sqrt : Sqrt
  Sqrt1 : Sqrt
  Square{1..4} (4 alike) : Math  Operator=square
  Step2 : Step  Time=0.01  SampleTime=Ts
  Step3 : Step  Time=0.01  SampleTime=Ts
  Sum6 : Sum  Inputs=|+-
  Sum9 : Sum  Inputs=|+-
  Switch1 : Switch  Threshold=.01  SaturateOnIntegerOverflow=off  InputSameDT=off
  Switch2 : Switch  Threshold=.01  SaturateOnIntegerOverflow=off  InputSameDT=off
  iubd : Outport
  iubq : Outport  Port=2
  wires:
  idref/1 -> Square4/1
  Sqrt1/1 -> iubq/1
  Imax/1 -> Square1/1, Square3/1
  Sqrt/1 -> iubd/1
  Constant9/1 -> Switch2/3
  Square4/1 -> Sum9/2
  Constant8/1 -> Switch1/3
  Square2/1 -> Sum6/2
  Sum6/1 -> Switch1/1
  Square3/1 -> Sum9/1
  iqref/1 -> Square2/1
  Switch1/1 -> Sqrt/1
  Square1/1 -> Sum6/1
  Switch2/1 -> Sqrt1/1
  Step2/1 -> Switch1/2
  Step3/1 -> Switch2/2
  Sum9/1 -> Switch2/1

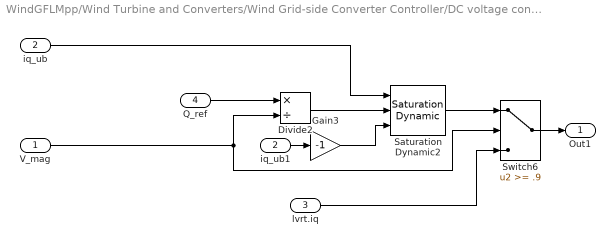
== system WindGFLMpp/Wind Turbine and Converters/Wind Grid-side Converter Controller/DC voltage controller & current reference/Subsystem ==
  V_mag : Inport
  iq_ub : Inport  Port=2
  lvrt.iq : Inport  Port=3
  Q_ref : Inport  Port=4
  Divide2 : Product  Inputs=*/
  Gain3 : Gain  Gain=-1
  Saturation Dynamic2 : simulink/Discontinuities/Saturation Dynamic  OutMin=[]  OutMax=[]  OutDataTypeStr=Inherit: Same as second input  OutDataType=fixdt(1, 16)  OutScaling=2^-10  DoSatur=off
  Switch6 : Switch  Threshold=.9  SaturateOnIntegerOverflow=off  InputSameDT=off
  iq_ub1 : InportShadow  Port=2
  Out1 : Outport
  wires:
  lvrt.iq/1 -> Switch6/3
  Switch6/1 -> Out1/1
  Saturation Dynamic2/1 -> Switch6/1
  iq_ub/1 -> Saturation Dynamic2/1
  Gain3/1 -> Saturation Dynamic2/3
  Q_ref/1 -> Divide2/1
  Divide2/1 -> Saturation Dynamic2/2
  iq_ub1/1 -> Gain3/1
  V_mag/1 -> Divide2/2, Switch6/2

== system WindGFLMpp/Wind Turbine and Converters/Wind Grid-side Converter Controller/DC voltage controller & current reference/Subsystem1 ==
  Wind_Mpp_vdc : Inport
  Wind_vdc : Inport  Port=2
  id_ub : Inport  Port=3
  Constant4 : Constant  Value=0
  Saturation Dynamic1 : simulink/Discontinuities/Saturation Dynamic  OutMin=[]  OutMax=[]  OutDataTypeStr=Inherit: Same as second input  OutDataType=fixdt(1, 16)  OutScaling=2^-10  DoSatur=off
  V_dc_Controller1 : Subsystem
  Out1 : Outport
  wires:
  Wind_Mpp_vdc/1 -> V_dc_Controller1/1(Wind_plant1)
  Saturation Dynamic1/1 -> Out1/1
  id_ub/1 -> Saturation Dynamic1/1
  Wind_vdc/1 -> V_dc_Controller1/2(In2)
  V_dc_Controller1/1(Out1) -> Saturation Dynamic1/2
  Constant4/1 -> Saturation Dynamic1/3

== system WindGFLMpp/Wind Turbine and Converters/Wind Grid-side Converter Controller/DC voltage controller & current reference/Subsystem1/V_dc_Controller1 ==
  Wind_plant1 : Inport
  In2 : Inport  Port=2
  Gain : Gain  Gain=1/windController.vdcBase
  PI : Subsystem
  Sum : Sum  Inputs=|+-
  Out1 : Outport
  wires:
  PI/1(Out2) -> Out1/1
  Gain/1 -> PI/1(Input)
  Sum/1 -> Gain/1
  In2/1 -> Sum/2
  Wind_plant1/1 -> Sum/1

== system WindGFLMpp/Wind Turbine and Converters/Wind Grid-side Converter Controller/DC voltage controller & current reference/Subsystem1/V_dc_Controller1/PI ==
  Input : Inport
  Discrete-Time Integrator : DiscreteIntegrator  gainval=Ki_dc  SampleTime=grid.sensorTime  ICPrevOutput=DiscIntNeverNeededParam  ICPrevScaledInput=DiscIntNeverNeededParam
  Gain1 : Gain  Gain=Kp_dc
  Sum1 : Sum  Inputs=|++
  Unit Delay : UnitDelay  SampleTime=grid.sensorTime  HasFrameUpgradeWarning=on
  Out2 : Outport
  wires:
  Input/1 -> Discrete-Time Integrator/1, Gain1/1
  Gain1/1 -> Unit Delay/1
  Unit Delay/1 -> Sum1/2
  Sum1/1 -> Out2/1
  Discrete-Time Integrator/1 -> Sum1/1
